simulink model "pulse_gen_model"  (R2018b)
settings: Solver=VariableStepAuto  StartTime=0.0  StopTime=Endtime  RelTol=1e-3
values from neighbouring files (symbols this model uses):
  alpha_P = 100/(2^m - 1)    (= 0.392156862745)    [controller_sim.m]    (also in pulse_gen_sim.m)
  d_P_d = 5    [controller_sim.m]    (also in pulse_gen_sim.m)
  m = 8    [controller_sim.m]    (also in pulse_gen_sim.m)
  smp = 0.001    [ADC_sim.m]    (also in controller_sim.m; pulse_gen_sim.m = 0.01)
libraries: simulink x1
settings Model: Creator=nharada  LastModifiedBy=nharada

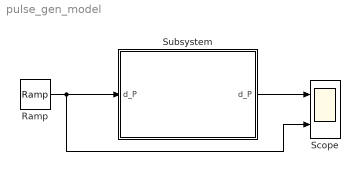
== system pulse_gen_model ==
  Ramp : simulink/Sources/Ramp  slope=d_P_d  start=0  InitialOutput=-50
  Scope : Scope  NumInputPorts=2
  Subsystem : Subsystem
  wires:
  Subsystem/1(d_P) -> Scope/1
  Ramp/1 -> Scope/2, Subsystem/1("d_P ")

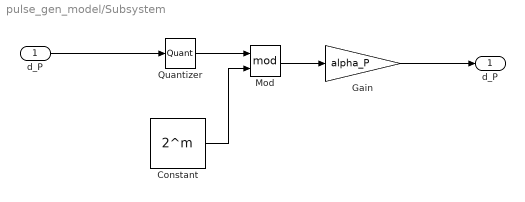
== system pulse_gen_model/Subsystem ==
  "d_P " : Inport
  Constant : Constant  Value=2^m  SampleTime=smp
  Gain : Gain  Gain=alpha_P
  Mod : Math  Operator=mod  SaturateOnIntegerOverflow=on
  Quantizer : Quantizer  QuantizationInterval=1
  d_P : Outport
  wires:
  Quantizer/1 -> Mod/1
  Constant/1 -> Mod/2
  Mod/1 -> Gain/1
  Gain/1 -> d_P/1
  "d_P "/1 -> Quantizer/1
